simulink model "SimpleHeloSim"  (R2021b)
settings: Solver=VariableStepAuto  StartTime=0.0  StopTime=15.  RelTol=1e-3
values from neighbouring files (symbols this model uses):
  u0 = [0;0;20.;25.]    [SimpleHeloInit.m]    (also in SimpleHeloInit_WW.m; SingleTrim.m; plot_AttitudeAndControlsAndEigenvalues.m = u0_vals(i,:)'; test.m)
  x0 = zeros(constants.NSTATES,1)    [SimpleHeloInit.m]    (also in SimpleHeloInit_WW.m; SingleTrim.m; plot_AttitudeAndControlsAndEigenvalues.m = x0_vals(i,:)'; test.m)
libraries: simulink x2
settings Model: Creator=jfh19  LastModifiedBy=Guowei
settings SolverCC: AlgebraicLoopSolver=TrustRegion
settings DataIOCC: ReturnWorkspaceOutputs=off
settings DebuggingCC: SFMachineParentedDataDiag=warning  ArithmeticOperatorsInVariantConditions=warning
settings SFSimCC: SimUseLocalCustomCode=off  CustomCodeUndefinedFunction=UseInterfaceOnly
settings RTWCC: RTWUseLocalCustomCode=off
settings CodeAppCC: StateflowObjectComments=on

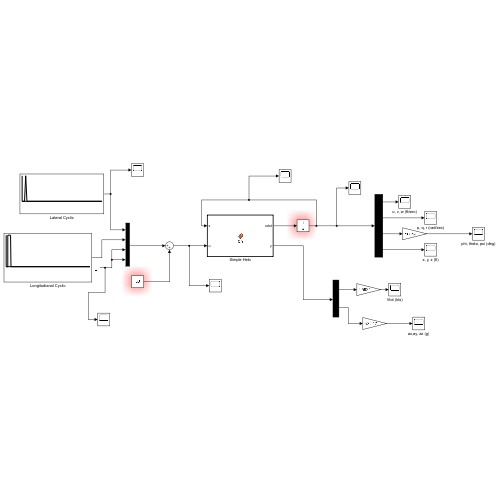
[thumbnail: Simulink's stored preview of the top-level diagram]
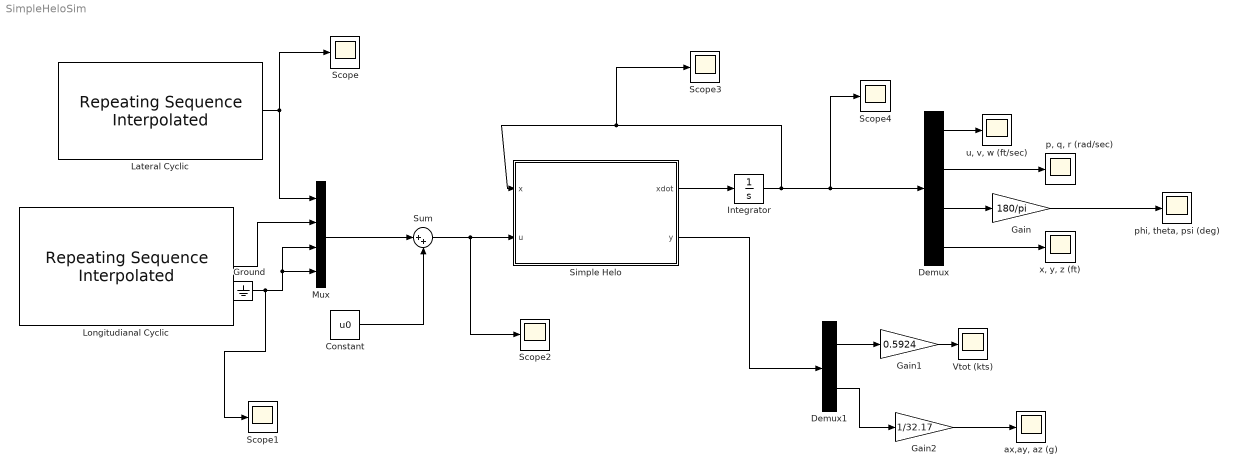
== system SimpleHeloSim ==
  Constant : Constant  Value=u0
  Demux : Demux  Outputs=[3;3;3;3]
  Demux1 : Demux  Outputs=[1;3]
  Gain : Gain  Gain=180/pi
  Gain1 : Gain  Gain=0.5924
  Gain2 : Gain  Gain=1/32.17
  Ground : Ground
  Integrator : Integrator  InitialCondition=x0
  Lateral Cyclic : simulink/Sources/Repeating Sequence Interpolated  OutValues=[0 0 0.1 0 0]  TimeValues=[0 1. 1.5 2.0 35.]  LookUpMeth=Interpolation-Use End Values  tsamp=0.01  OutMin=[]  OutMax=[]  OutDataTypeStr=double  OutputDataTypeScalingMode=double  OutDataType=fixdt(0,8)  OutScaling=2^-10
  Longitudianal Cyclic : simulink/Sources/Repeating Sequence Interpolated  OutValues=[0 0 0.5 0.5 0 0].'  TimeValues=[0 1 1.1 3.1 3.2 60].'  LookUpMeth=Interpolation-Use End Values  tsamp=0.01  OutMin=[]  OutMax=[]  OutDataTypeStr=double  OutputDataTypeScalingMode=double  OutDataType=fixdt(0,8)  OutScaling=2^-10
  Mux : Mux
  Scope{,1..4} (5 alike) : Scope
  Simple Helo : MATLAB Function  TreatAsAtomicUnit=on
  Sum : Sum  Inputs=|++
  Vtot (kts) : Scope
  "ax,ay, az (g)" : Scope
  "p, q, r (rad/sec)" : Scope
  "phi, theta, psi (deg)" : Scope
  "u, v, w (ft/sec)" : Scope
  "x, y, z (ft)" : Scope
  wires:
  Simple Helo/1(xdot) -> Integrator/1
  Integrator/1 -> Scope4/1, Demux/1, Scope3/1, Simple Helo/1(x)
  Demux/1 -> "u, v, w (ft/sec)"/1
  Demux/2 -> "p, q, r (rad/sec)"/1
  Demux/3 -> Gain/1
  Demux/4 -> "x, y, z (ft)"/1
  Sum/1 -> Scope2/1, Simple Helo/2(u)
  Constant/1 -> Sum/2
  Mux/1 -> Sum/1
  Ground/1 -> Scope1/1, Mux/3, Mux/4
  Lateral Cyclic/1 -> Mux/1, Scope/1
  Simple Helo/2(y) -> Demux1/1
  Demux1/2 -> Gain2/1
  Demux1/1 -> Gain1/1
  Gain/1 -> "phi, theta, psi (deg)"/1
  Gain1/1 -> Vtot (kts)/1
  Gain2/1 -> "ax,ay, az (g)"/1
  Longitudianal Cyclic/1 -> Mux/2

== matlab function SimpleHeloSim/Simple Helo ==
  data: x input size=constants.NSTATES; xdot output; u input size=constants.NCTRLS; y output size=constants.NOUT; constants parameter
function [xdot,y] = fcn(x,u,constants)
%eml
% Interesting, the state vector x for the simulation is 0 at the beginning.
[xdot,y] = SimpleHelo(x,u,[],constants);
